simulink model "disturbance_observers"  (R2015a)
settings: Solver=ode45  StartTime=0.0  StopTime=10.0  RelTol=1e-3
undefined symbols (not defined in the file or in its folder): g, i_robot, L_dob_xdx_thetadtheta, L_dob_zdz, m_total_real, sample_time
settings Model: Creator=wmartin  LastModifiedBy=wmartin

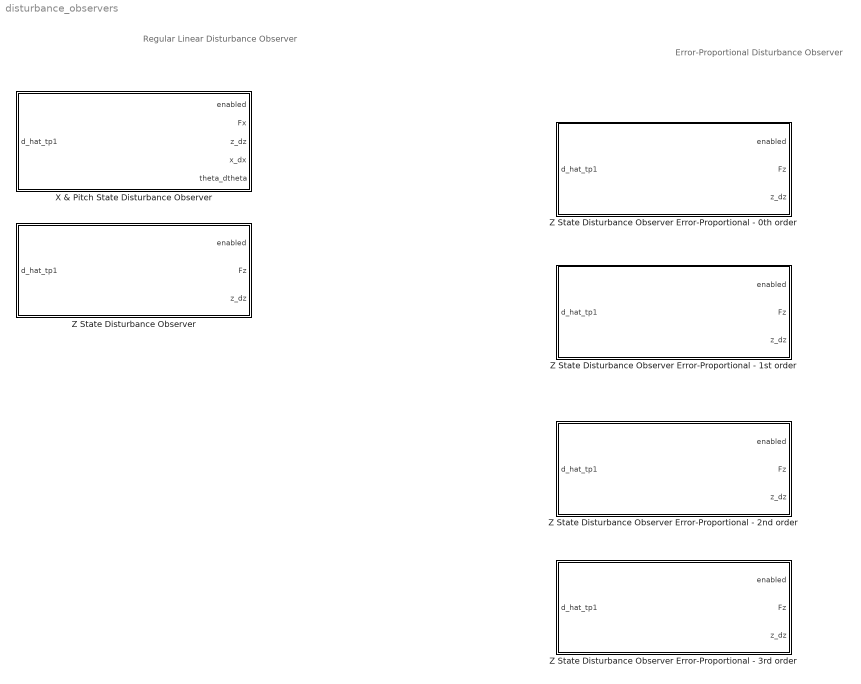
== system disturbance_observers ==
  note: Regular Linear Disturbance Observer
  note: Error-Proportional Disturbance Observer
  X & Pitch State Disturbance Observer : MATLAB Function  TreatAsAtomicUnit=on
  Z State Disturbance Observer : MATLAB Function  TreatAsAtomicUnit=on
  Z State Disturbance Observer Error-Proportional - 0th order : MATLAB Function  TreatAsAtomicUnit=on
  Z State Disturbance Observer Error-Proportional - 1st order : MATLAB Function  TreatAsAtomicUnit=on
  Z State Disturbance Observer Error-Proportional - 2nd order : MATLAB Function  TreatAsAtomicUnit=on
  Z State Disturbance Observer Error-Proportional - 3rd order : MATLAB Function  TreatAsAtomicUnit=on

== matlab function disturbance_observers/X & Pitch State Disturbance Observer ==
  data: enabled input; Fx input size=1; z_dz input; d_hat_tp1 output size=1; x_dx input size=2; theta_dtheta input; L_dob_xdx_thetadtheta parameter; sample_time parameter; m_total_real parameter; g parameter; i_robot parameter
function d_hat_tp1 = disturbance_observer(enabled, Fx, z_dz, x_dx, theta_dtheta, L_dob_xdx_thetadtheta, sample_time, m_total_real, g, i_robot)

    persistent z_t;
    if isempty(z_t) || enabled
        z_t = 0;
    end

    % Define system
    A_d = [ 1, 0, sample_time, 0;
            0, 1, 0, sample_time;
            0, 0, 1, 0;
            m_total_real*g*sample_time/i_robot, 0, 0, 1];
    Bu_d = [0; 0; sample_time/m_total_real; -sample_time*z_dz(1)/i_robot];
    A_c = [ 0, 0, 1, 0;
            0, 0, 0, 1;
            0, 0, 0, 0;
            m_total_real*g/i_robot, 0, 0, 0];
    Bu_c = [0; 0; 1/m_total_real; -z_dz(1)/i_robot];
    Bd_c = [0; 0; 1/m_total_real; -z_dz(1)/i_robot];
    L = L_dob_xdx_thetadtheta;
    x = [x_dx(1); theta_dtheta(1); x_dx(2); theta_dtheta(2)];
    u = Fx;

    % Estimate disturbance
    x_tp1 = A_d*x + Bu_d*u;
    z_tp1 = z_t - sample_time*L*(Bd_c*(z_t + L*x) + A_c*x + Bu_c*u);
    d_hat_tp1 = z_tp1 + L*x_tp1;
    z_t = z_tp1;

end

== matlab function disturbance_observers/Z State Disturbance Observer ==
  data: enabled input; Fz input size=1; d_hat_tp1 output size=1; z_dz input size=2; L_dob_zdz parameter; m_total_real parameter; g parameter; sample_time parameter
function d_hat_tp1  = disturbance_observer(enabled, Fz, z_dz, L_dob_zdz, m_total_real, g, sample_time)

    persistent z_t;
    if isempty(z_t) || enabled
        z_t = 0;
    end
    
    % Define system
    A_d = [1, sample_time; 0, 1];
    Bu_d = [0; sample_time/m_total_real];
    A_c = [0 1; 0 0];
    Bu_c = [0; 1/m_total_real];
    Bd_c = [0; 1/m_total_real];
    L = L_dob_zdz;
    x = z_dz;
    u = Fz - m_total_real*g;
    
    % Estimate disturbance
    x_tp1 = A_d*x + Bu_d*u;
    z_tp1 = z_t - sample_time*L*(Bd_c*(z_t + L*x) + A_c*x + Bu_c*u);
    d_hat_tp1 = z_tp1 + L*x_tp1;
    z_t = z_tp1;
    
end

== matlab function disturbance_observers/Z State Disturbance Observer Error-Proportional - 0th order ==
  data: enabled input; Fz input size=1; d_hat_tp1 output size=1; z_dz input size=2; L_dob_zdz parameter; m_total_real parameter; g parameter; sample_time parameter
function d_hat_tp1  = disturbance_observer(enabled, Fz, z_dz, L_dob_zdz, m_total_real, g, sample_time)

    persistent z_t;
    if isempty(z_t) || enabled
        z_t = 0;
    end
    
    persistent d_hat_t;
    if isempty(d_hat_t) || enabled
        d_hat_t = 0;
    end
    
    % Define system
    A_d = [1, sample_time; 0, 1];
    Bu_d = [0; sample_time/m_total_real];
    A_c = [0 1; 0 0];
    Bu_c = [0; 1/m_total_real];
    Bd_c = [0; 1/m_total_real];
    L = 2;
    x = z_dz;
    u = Fz - m_total_real*g;
    
    % Estimate disturbance
    z_tp1 = z_t + sample_time*(pinv(Bd_c)*(A_c*x + Bu_c*u) + d_hat_t);
    x_tp1 = A_d*x + Bu_d*u;
    d_hat_tp1 = L*(pinv(Bd_c)*x_tp1 - z_tp1);
    d_hat_t = d_hat_tp1;
    z_t = z_tp1;
    
end

== matlab function disturbance_observers/Z State Disturbance Observer Error-Proportional - 1st order ==
  data: enabled input; Fz input size=1; d_hat_tp1 output size=1; z_dz input size=2; L_dob_zdz parameter; m_total_real parameter; g parameter; sample_time parameter
function d_hat_tp1  = disturbance_observer(enabled, Fz, z_dz, L_dob_zdz, m_total_real, g, sample_time)

    persistent z_t;
    if isempty(z_t) || enabled
        z_t = 0;
    end
    
    persistent d_hat_t;
    if isempty(d_hat_t) || enabled
        d_hat_t = 0;
    end
    
    persistent integral_term;
    if isempty(integral_term) || enabled
        integral_term = 0;
    end
    
    % Define system
    A_d = [1, sample_time; 0, 1];
    Bu_d = [0; sample_time/m_total_real];
    A_c = [0 1; 0 0];
    Bu_c = [0; 1/m_total_real];
    Bd_c = [0; 1/m_total_real];
    L = [4, 4];
    x = z_dz;
    u = Fz - m_total_real*g;
    
    % Estimate disturbance
    z_tp1 = z_t + sample_time*(pinv(Bd_c)*(A_c*x + Bu_c*u) + d_hat_t);
    x_tp1 = A_d*x + Bu_d*u;
    integral_term = integral_term + sample_time*(pinv(Bd_c)*x_tp1 - z_tp1);
    d_hat_tp1 = L(1)*(pinv(Bd_c)*x_tp1 - z_tp1) + L(2)*integral_term;
    d_hat_t = d_hat_tp1;
    z_t = z_tp1;
    
end

== matlab function disturbance_observers/Z State Disturbance Observer Error-Proportional - 2nd order ==
  data: enabled input; Fz input size=1; d_hat_tp1 output size=1; z_dz input size=2; L_dob_zdz parameter; m_total_real parameter; g parameter; sample_time parameter
function d_hat_tp1  = disturbance_observer(enabled, Fz, z_dz, L_dob_zdz, m_total_real, g, sample_time)

    persistent z_t;
    if isempty(z_t) || enabled
        z_t = 0;
    end
    
    persistent d_hat_t;
    if isempty(d_hat_t) || enabled
        d_hat_t = 0;
    end
    
    persistent integral_term;
    if isempty(integral_term) || enabled
        integral_term = [0, 0];
    end
    
    % Define system
    A_d = [1, sample_time; 0, 1];
    Bu_d = [0; sample_time/m_total_real];
    A_c = [0 1; 0 0];
    Bu_c = [0; 1/m_total_real];
    Bd_c = [0; 1/m_total_real];
    L = [6, 12, 8];
    x = z_dz;
    u = Fz - m_total_real*g;
    
    % Estimate disturbance
    z_tp1 = z_t + sample_time*(pinv(Bd_c)*(A_c*x + Bu_c*u) + d_hat_t);
    x_tp1 = A_d*x + Bu_d*u;
    integral_term(1) = integral_term(1) + sample_time*(pinv(Bd_c)*x_tp1 - z_tp1);
    integral_term(2) = integral_term(2) + sample_time*integral_term(1);
    d_hat_tp1 = L(1)*(pinv(Bd_c)*x_tp1 - z_tp1) + L(2)*integral_term(1) + L(3)*integral_term(2);
    d_hat_t = d_hat_tp1;
    z_t = z_tp1;
    
end

== matlab function disturbance_observers/Z State Disturbance Observer Error-Proportional - 3rd order ==
  data: enabled input; Fz input size=1; d_hat_tp1 output size=1; z_dz input size=2; L_dob_zdz parameter; m_total_real parameter; g parameter; sample_time parameter
function d_hat_tp1  = disturbance_observer(enabled, Fz, z_dz, L_dob_zdz, m_total_real, g, sample_time)

    order = 3;
    L = 2.^[1:order+1] .* factorial(order+1)./(factorial(order+1-(1:(order+1))).*factorial(1:order+1));

    persistent z_t d_hat_t integral_term;
    if isempty(z_t) || enabled
        z_t = 0;
        d_hat_t = 0;
        integral_term = zeros(order,1);
    end
   
    % Define system
    A_d = [1, sample_time; 0, 1];
    Bu_d = [0; sample_time/m_total_real];
    A_c = [0 1; 0 0];
    Bu_c = [0; 1/m_total_real];
    Bd_c = [0; 1/m_total_real];
    x = z_dz;
    u = Fz - m_total_real*g;
 
    % Estimate disturbance
    z_tp1 = z_t + sample_time*(pinv(Bd_c)*(A_c*x + Bu_c*u) + d_hat_t);
    x_tp1 = A_d*x + Bu_d*u;
    integral_term(1) = integral_term(1) + sample_time*(pinv(Bd_c)*x_tp1 - z_tp1);
    for i=2:order
        integral_term(i) = integral_term(i) + sample_time*integral_term(i-1);
    end
    d_hat_tp1 = L*[(pinv(Bd_c)*x_tp1 - z_tp1); integral_term];
    d_hat_t = d_hat_tp1;
    z_t = z_tp1;
    
end
